simulink model "MultiDOFSystem"  (R2020a)
settings: Solver=FixedStepAuto  StartTime=0.0  StopTime=170  FixedStep=.08  RelTol=1e-3
model workspace (MAT data in the model file):
  c1 = Simulink.Parameter
  c1.Value = 11
  c1.DataType = 'auto'
  c1.DocUnits = 'Ns/m'
  c1.Dimensions = [1 1]
  c2 = Simulink.Parameter
  c2.Value = 11
  c2.DataType = 'auto'
  c2.DocUnits = 'Ns/m'
  c2.Dimensions = [1 1]
  c3 = Simulink.Parameter
  c3.Value = 11
  c3.DataType = 'auto'
  c3.DocUnits = 'Ns/m'
  c3.Dimensions = [1 1]
  k1 = Simulink.Parameter
  k1.Value = 50
  k1.DataType = 'auto'
  k1.DocUnits = 'N/m'
  k1.Dimensions = [1 1]
  k2 = Simulink.Parameter
  k2.Value = 50
  k2.DataType = 'auto'
  k2.DocUnits = 'N/m'
  k2.Dimensions = [1 1]
  k3 = Simulink.Parameter
  k3.Value = 50
  k3.DataType = 'auto'
  k3.DocUnits = 'N/m'
  k3.Dimensions = [1 1]
  m1 = Simulink.Parameter
  m1.Value = 5
  m1.DataType = 'auto'
  m1.DocUnits = 'kg'
  m1.Dimensions = [1 1]
  m2 = Simulink.Parameter
  m2.Value = 5
  m2.DataType = 'auto'
  m2.DocUnits = 'kg'
  m2.Dimensions = [1 1]
  m3 = Simulink.Parameter
  m3.Value = 5
  m3.DataType = 'auto'
  m3.DocUnits = 'kg'
  m3.Dimensions = [1 1]
settings Model: Creator=13ann  LastModifiedBy=13ann

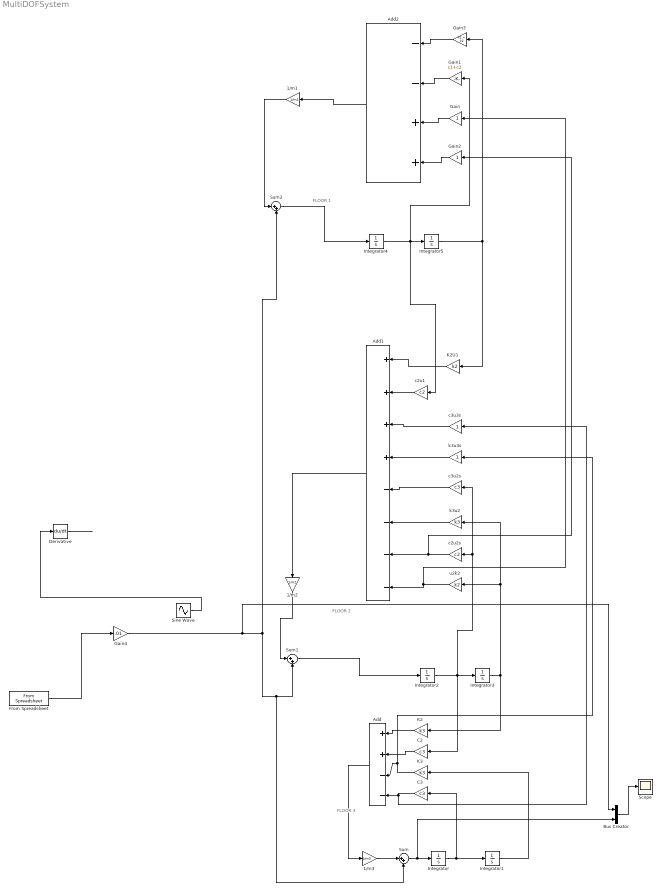
== system MultiDOFSystem ==
  note: FLOOR 1
  note: FLOOR 2
  note: FLOOR 3
  "\tK2" : Gain  Gain=k3
  "\tK2U1" : Gain  Gain=k2
  1/m1 : Gain  Gain=1/m1
  1/m2 : Gain  Gain=1/m2
  1/m3 : Gain  Gain=1/m3
  Add : Sum  Inputs=++--
  Add1 : Sum  Inputs=++++----
  Add2 : Sum  Inputs=--++
  Bus Creator : BusCreator  Inputs=2
  C2 : Gain  Gain=c3
  C3 : Gain  Gain=c3
  Derivative : Derivative
  From Spreadsheet : FromSpreadsheet  FileName=Book1.xlsx  Range=D1:D2150  TreatFirstColumnAs=Data  SampleTime=.08
  Gain : Gain
  Gain1 : Gain  Gain=c1+c2
  Gain2 : Gain
  Gain3 : Gain  Gain=k1 + k2
  Gain4 : Gain  Gain=.01
  Integrator{,1..5} (6 alike) : Integrator
  K3 : Gain  Gain=k3
  Scope : Scope
  Sine Wave : Sin  Amplitude=0.02  SampleTime=0
  Sum : Sum  Inputs=|++
  Sum1 : Sum  Inputs=|++
  Sum2 : Sum  Inputs=|++
  c2u1 : Gain  Gain=c2
  c2u2s : Gain  Gain=c2
  c3u2s : Gain  Gain=c3
  c3u3s : Gain
  k3u2 : Gain  Gain=k3
  k3u3s : Gain
  u2k2 : Gain  Gain=k2
  wires:
  Integrator/1 -> Integrator1/1, C3/1
  Integrator1/1 -> K3/1
  Integrator2/1 -> c3u2s/1, c2u2s/1, Integrator3/1, C2/1
  Integrator3/1 -> k3u2/1, u2k2/1, "\tK2"/1
  Integrator4/1 -> Gain1/1, c2u1/1, Integrator5/1
  Integrator5/1 -> "\tK2U1"/1, Gain3/1
  K3/1 -> k3u3s/1, Add/3
  C3/1 -> c3u3s/1, Add/4
  Add/1 -> 1/m3/1
  "\tK2"/1 -> Add/1
  C2/1 -> Add/2
  "\tK2U1"/1 -> Add1/1
  u2k2/1 -> Gain/1, Add1/8
  c2u2s/1 -> Gain2/1, Add1/7
  k3u2/1 -> Add1/6
  c3u2s/1 -> Add1/5
  c2u1/1 -> Add1/2
  c3u3s/1 -> Add1/3
  k3u3s/1 -> Add1/4
  Add1/1 -> 1/m2/1
  Gain2/1 -> Add2/4
  Gain/1 -> Add2/3
  Gain1/1 -> Add2/2
  Gain3/1 -> Add2/1
  Add2/1 -> 1/m1/1
  Sine Wave/1 -> Derivative/1
  Derivative/1 -> ?
  1/m3/1 -> Sum/1
  Sum/1 -> Bus Creator/2, Integrator/1
  Sum1/1 -> Integrator2/1
  1/m2/1 -> Sum1/1
  1/m1/1 -> Sum2/1
  Sum2/1 -> Integrator4/1
  Gain4/1 -> Bus Creator/1, Sum1/2, Sum/2, Sum2/2
  From Spreadsheet/1 -> Gain4/1
  Bus Creator/1 -> Scope/1
